simulink model "FinalSim"  (R2022b)
settings: Solver=VariableStepAuto  StartTime=0.0  StopTime=10  RelTol=1e-3
libraries: eeGeneralControl x3
(part 5 of 7)

== system FinalSim/Shoulder Adductor Model/Shoulder Transverse Flexors1/fascicles (CE & PE)/Type S Motor Units ==
  fenv : Inport
  V,L : Inport  Port=2
  Fpe2 : Inport  Port=3
  1/Ty : Gain  Gain=5  SaturateOnIntegerOverflow=on  OutDataTypeStr=Inherit: Same as input  ParamDataTypeStr=Inherit: Same as input
  Af*(FL*FV+PE2) : Product  InputSameDT=on  RndMeth=Zero  SaturateOnIntegerOverflow=on  OutDataTypeStr=Inherit: Same as first input
  Demux all Units : Demux  Outputs=2
      settings: DisplayOption=none
  FL : Fcn  Expr=exp(-abs((u^2.3-1)/1.1244)^1.62)
  FL*FV : Product  InputSameDT=on  RndMeth=Zero  SaturateOnIntegerOverflow=on  OutDataTypeStr=Inherit: Same as first input
  FV (lengthen) : Fcn  Expr=(0.34936-(-4.7+8.41*u(2)+-5.31*u(2)^2)*u(1))/(0.34936+u(1))
  FV (shorten) : Fcn  Expr=(-7.88-u(1))/(-7.88+(5.88+0*u(2))*u(1))
  Motor Unit 1 : Subsystem
  Motor Unit 2 : Subsystem
  PCSA 1 : Gain  Gain=0.21429  SaturateOnIntegerOverflow=on  OutDataTypeStr=Inherit: Same as input  ParamDataTypeStr=Inherit: Same as input
  PCSA 2 : Gain  Gain=0.28571  SaturateOnIntegerOverflow=on  OutDataTypeStr=Inherit: Same as input  ParamDataTypeStr=Inherit: Same as input
  PE+FL*FV : Sum  InputSameDT=on  SaturateOnIntegerOverflow=on  OutDataTypeStr=Inherit: Same as first input
  Sum all Units : Sum  InputSameDT=on  SaturateOnIntegerOverflow=on  OutDataTypeStr=Inherit: Same as first input
  Y,L : Mux  Inputs=2
  newY-oldY : Sum  Inputs=+-  InputSameDT=on  SaturateOnIntegerOverflow=on  OutDataTypeStr=Inherit: Same as first input
  split V,L : Demux  Outputs=2
      settings: DisplayOption=none
  v > 0? : Switch
  y'->y : Integrator  InitialCondition=1
  yield : Fcn  Expr=1-0.35*(1-exp(-abs(u)/0.1))
  F (Fo) : Outport
  wires:
  split V,L/1 -> yield/1, v > 0?/2
  yield/1 -> newY-oldY/1
  newY-oldY/1 -> 1/Ty/1
  1/Ty/1 -> y'->y/1
  y'->y/1 -> newY-oldY/2, Y,L/1
  Y,L/1 -> Motor Unit 1/2(Y,L), Motor Unit 2/2(Y,L)
  Demux all Units/1 -> Motor Unit 1/1(fenv)
  Motor Unit 1/1(A) -> PCSA 1/1
  PCSA 1/1 -> Sum all Units/1
  Demux all Units/2 -> Motor Unit 2/1(fenv)
  Motor Unit 2/1(A) -> PCSA 2/1
  PCSA 2/1 -> Sum all Units/2
  Fpe2/1 -> PE+FL*FV/1
  V,L/1 -> FV (lengthen)/1, FV (shorten)/1, split V,L/1
  FV (lengthen)/1 -> v > 0?/1
  FV (shorten)/1 -> v > 0?/3
  split V,L/2 -> FL/1, Y,L/2
  FL/1 -> FL*FV/2
  v > 0?/1 -> FL*FV/1
  FL*FV/1 -> PE+FL*FV/2
  PE+FL*FV/1 -> Af*(FL*FV+PE2)/1
  fenv/1 -> Demux all Units/1
  Sum all Units/1 -> Af*(FL*FV+PE2)/2
  Af*(FL*FV+PE2)/1 -> F (Fo)/1

== system FinalSim/Shoulder Extensor/fascicles (CE & PE)/Type F Motor Units/Motor Unit 1 ==
  fenv : Inport
  Y,L : Inport  Port=2
  1/Tf (feff' < 0) : Fcn  Expr=u(2)/(0.02822+0.01513*u(3))
  1/Tf (feff' > 0) : Fcn  Expr=1/(0.02057*u(2)^2+0.0136*u(4))
  1/Ts : Gain  Gain=23.2558  SaturateOnIntegerOverflow=on  OutDataTypeStr=Inherit: Same as input  ParamDataTypeStr=Inherit: Same as input
  Af : Fcn  Expr=1-exp(-(u(1)*u(4)*u(3)/(0.56*u(2)))^u(2))
  Leff' : Fcn  Expr=(u(2)-u(1))^3/((1-u(3))*8.8e-005)
  Leff'->Leff : Integrator  InitialCondition=1
  "Leff,L, Af,fenv" : Mux
  S and old S diff : Sum  Inputs=-+  InputSameDT=on  SaturateOnIntegerOverflow=on  OutDataTypeStr=Inherit: Same as first input
  Y,nf,feff,S : Mux
  aS1 : Constant  Value=1.76
  aS2 : Constant  Value=0.96
  demux Y,L : Demux  Outputs=2
      settings: DisplayOption=none
  feff' : Product  InputSameDT=on  RndMeth=Zero  SaturateOnIntegerOverflow=on  OutDataTypeStr=Inherit: Same as first input
  feff' > 0? : Switch
  feff'->feff : Integrator
  feff>0.1? : Switch  Threshold=0.1
  fenv-fint : Sum  Inputs=+-  InputSameDT=on  SaturateOnIntegerOverflow=on  OutDataTypeStr=Inherit: Same as first input
  fint' : Product  InputSameDT=on  RndMeth=Zero  SaturateOnIntegerOverflow=on  OutDataTypeStr=Inherit: Same as first input
  fint'->fint : Integrator
  fint-feff : Sum  Inputs=+-  InputSameDT=on  SaturateOnIntegerOverflow=on  OutDataTypeStr=Inherit: Same as first input
  nf : Fcn  Expr=2.11+3.31*(1/u-1)
  s'->s : Integrator  InitialCondition=1.76
  A : Outport
  wires:
  Y,L/1 -> demux Y,L/1
  demux Y,L/1 -> Y,nf,feff,S/1
  demux Y,L/2 -> "Leff,L, Af,fenv"/2
  "Leff,L, Af,fenv"/1 -> 1/Tf (feff' < 0)/1, Leff'/1, 1/Tf (feff' > 0)/1
  1/Tf (feff' > 0)/1 -> feff' > 0?/1
  1/Tf (feff' < 0)/1 -> feff' > 0?/3
  fenv/1 -> fenv-fint/1, "Leff,L, Af,fenv"/4
  fenv-fint/1 -> fint'/2
  fint'/1 -> fint'->fint/1
  fint'->fint/1 -> fint-feff/1, fenv-fint/2
  fint-feff/1 -> feff'/2, feff' > 0?/2
  feff' > 0?/1 -> feff'/1, fint'/1
  feff'/1 -> feff'->feff/1
  feff'->feff/1 -> fint-feff/2, Y,nf,feff,S/3, feff>0.1?/2
  Y,nf,feff,S/1 -> Af/1
  Af/1 -> "Leff,L, Af,fenv"/3, A/1
  Leff'/1 -> Leff'->Leff/1
  Leff'->Leff/1 -> "Leff,L, Af,fenv"/1, nf/1
  nf/1 -> Y,nf,feff,S/2
  aS2/1 -> feff>0.1?/1
  aS1/1 -> feff>0.1?/3
  feff>0.1?/1 -> S and old S diff/2
  S and old S diff/1 -> 1/Ts/1
  1/Ts/1 -> s'->s/1
  s'->s/1 -> S and old S diff/1, Y,nf,feff,S/4

== system FinalSim/Shoulder Extensor/fascicles (CE & PE)/Type F Motor Units/Motor Unit 2 ==
  fenv : Inport
  Y,L : Inport  Port=2
  1/Tf (feff' < 0) : Fcn  Expr=u(2)/(0.02822+0.01513*u(3))
  1/Tf (feff' > 0) : Fcn  Expr=1/(0.02057*u(2)^2+0.0136*u(4))
  1/Ts : Gain  Gain=23.2558  SaturateOnIntegerOverflow=on  OutDataTypeStr=Inherit: Same as input  ParamDataTypeStr=Inherit: Same as input
  Af : Fcn  Expr=1-exp(-(u(1)*u(4)*u(3)/(0.56*u(2)))^u(2))
  Leff' : Fcn  Expr=(u(2)-u(1))^3/((1-u(3))*8.8e-005)
  Leff'->Leff : Integrator  InitialCondition=1
  "Leff,L, Af,fenv" : Mux
  S and old S diff : Sum  Inputs=-+  InputSameDT=on  SaturateOnIntegerOverflow=on  OutDataTypeStr=Inherit: Same as first input
  Y,nf,feff,S : Mux
  aS1 : Constant  Value=1.76
  aS2 : Constant  Value=0.96
  demux Y,L : Demux  Outputs=2
      settings: DisplayOption=none
  feff' : Product  InputSameDT=on  RndMeth=Zero  SaturateOnIntegerOverflow=on  OutDataTypeStr=Inherit: Same as first input
  feff' > 0? : Switch
  feff'->feff : Integrator
  feff>0.1? : Switch  Threshold=0.1
  fenv-fint : Sum  Inputs=+-  InputSameDT=on  SaturateOnIntegerOverflow=on  OutDataTypeStr=Inherit: Same as first input
  fint' : Product  InputSameDT=on  RndMeth=Zero  SaturateOnIntegerOverflow=on  OutDataTypeStr=Inherit: Same as first input
  fint'->fint : Integrator
  fint-feff : Sum  Inputs=+-  InputSameDT=on  SaturateOnIntegerOverflow=on  OutDataTypeStr=Inherit: Same as first input
  nf : Fcn  Expr=2.11+3.31*(1/u-1)
  s'->s : Integrator  InitialCondition=1.76
  A : Outport
  wires:
  Y,L/1 -> demux Y,L/1
  demux Y,L/1 -> Y,nf,feff,S/1
  demux Y,L/2 -> "Leff,L, Af,fenv"/2
  "Leff,L, Af,fenv"/1 -> 1/Tf (feff' < 0)/1, Leff'/1, 1/Tf (feff' > 0)/1
  1/Tf (feff' > 0)/1 -> feff' > 0?/1
  1/Tf (feff' < 0)/1 -> feff' > 0?/3
  fenv/1 -> fenv-fint/1, "Leff,L, Af,fenv"/4
  fenv-fint/1 -> fint'/2
  fint'/1 -> fint'->fint/1
  fint'->fint/1 -> fint-feff/1, fenv-fint/2
  fint-feff/1 -> feff'/2, feff' > 0?/2
  feff' > 0?/1 -> feff'/1, fint'/1
  feff'/1 -> feff'->feff/1
  feff'->feff/1 -> fint-feff/2, Y,nf,feff,S/3, feff>0.1?/2
  Y,nf,feff,S/1 -> Af/1
  Af/1 -> "Leff,L, Af,fenv"/3, A/1
  Leff'/1 -> Leff'->Leff/1
  Leff'->Leff/1 -> "Leff,L, Af,fenv"/1, nf/1
  nf/1 -> Y,nf,feff,S/2
  aS2/1 -> feff>0.1?/1
  aS1/1 -> feff>0.1?/3
  feff>0.1?/1 -> S and old S diff/2
  S and old S diff/1 -> 1/Ts/1
  1/Ts/1 -> s'->s/1
  s'->s/1 -> S and old S diff/1, Y,nf,feff,S/4

== system FinalSim/Shoulder Extensor/fascicles (CE & PE)/Type F Motor Units/Motor Unit 3 ==
  fenv : Inport
  Y,L : Inport  Port=2
  1/Tf (feff' < 0) : Fcn  Expr=u(2)/(0.02822+0.01513*u(3))
  1/Tf (feff' > 0) : Fcn  Expr=1/(0.02057*u(2)^2+0.0136*u(4))
  1/Ts : Gain  Gain=23.2558  SaturateOnIntegerOverflow=on  OutDataTypeStr=Inherit: Same as input  ParamDataTypeStr=Inherit: Same as input
  Af : Fcn  Expr=1-exp(-(u(1)*u(4)*u(3)/(0.56*u(2)))^u(2))
  Leff' : Fcn  Expr=(u(2)-u(1))^3/((1-u(3))*8.8e-005)
  Leff'->Leff : Integrator  InitialCondition=1
  "Leff,L, Af,fenv" : Mux
  S and old S diff : Sum  Inputs=-+  InputSameDT=on  SaturateOnIntegerOverflow=on  OutDataTypeStr=Inherit: Same as first input
  Y,nf,feff,S : Mux
  aS1 : Constant  Value=1.76
  aS2 : Constant  Value=0.96
  demux Y,L : Demux  Outputs=2
      settings: DisplayOption=none
  feff' : Product  InputSameDT=on  RndMeth=Zero  SaturateOnIntegerOverflow=on  OutDataTypeStr=Inherit: Same as first input
  feff' > 0? : Switch
  feff'->feff : Integrator
  feff>0.1? : Switch  Threshold=0.1
  fenv-fint : Sum  Inputs=+-  InputSameDT=on  SaturateOnIntegerOverflow=on  OutDataTypeStr=Inherit: Same as first input
  fint' : Product  InputSameDT=on  RndMeth=Zero  SaturateOnIntegerOverflow=on  OutDataTypeStr=Inherit: Same as first input
  fint'->fint : Integrator
  fint-feff : Sum  Inputs=+-  InputSameDT=on  SaturateOnIntegerOverflow=on  OutDataTypeStr=Inherit: Same as first input
  nf : Fcn  Expr=2.11+3.31*(1/u-1)
  s'->s : Integrator  InitialCondition=1.76
  A : Outport
  wires:
  Y,L/1 -> demux Y,L/1
  demux Y,L/1 -> Y,nf,feff,S/1
  demux Y,L/2 -> "Leff,L, Af,fenv"/2
  "Leff,L, Af,fenv"/1 -> 1/Tf (feff' < 0)/1, Leff'/1, 1/Tf (feff' > 0)/1
  1/Tf (feff' > 0)/1 -> feff' > 0?/1
  1/Tf (feff' < 0)/1 -> feff' > 0?/3
  fenv/1 -> fenv-fint/1, "Leff,L, Af,fenv"/4
  fenv-fint/1 -> fint'/2
  fint'/1 -> fint'->fint/1
  fint'->fint/1 -> fint-feff/1, fenv-fint/2
  fint-feff/1 -> feff'/2, feff' > 0?/2
  feff' > 0?/1 -> feff'/1, fint'/1
  feff'/1 -> feff'->feff/1
  feff'->feff/1 -> fint-feff/2, Y,nf,feff,S/3, feff>0.1?/2
  Y,nf,feff,S/1 -> Af/1
  Af/1 -> "Leff,L, Af,fenv"/3, A/1
  Leff'/1 -> Leff'->Leff/1
  Leff'->Leff/1 -> "Leff,L, Af,fenv"/1, nf/1
  nf/1 -> Y,nf,feff,S/2
  aS2/1 -> feff>0.1?/1
  aS1/1 -> feff>0.1?/3
  feff>0.1?/1 -> S and old S diff/2
  S and old S diff/1 -> 1/Ts/1
  1/Ts/1 -> s'->s/1
  s'->s/1 -> S and old S diff/1, Y,nf,feff,S/4

== system FinalSim/Shoulder Extensor/fascicles (CE & PE)/Type S Motor Units/Motor Unit 1 ==
  fenv : Inport
  Y,L : Inport  Port=2
  1/Tf (feff' < 0) : Fcn  Expr=u(2)/(0.047033+0.025217*u(3))
  1/Tf (feff' > 0) : Fcn  Expr=1/(0.034283*u(2)^2+0.022667*u(4))
  Af : Fcn  Expr=1-exp(-(u(1)*u(4)*u(3)/(0.56*u(2)))^u(2))
  Leff' : Fcn  Expr=(u(2)-u(1))^3/((1-u(3))*8.8e-005)
  Leff'->Leff : Integrator  InitialCondition=1
  "Leff,L, Af,fenv" : Mux
  Y,nf,feff,S : Mux
  aS : Constant
  demux Y,L : Demux  Outputs=2
      settings: DisplayOption=none
  feff' : Product  InputSameDT=on  RndMeth=Zero  SaturateOnIntegerOverflow=on  OutDataTypeStr=Inherit: Same as first input
  feff' > 0? : Switch
  feff'->feff : Integrator
  fenv-fint : Sum  Inputs=+-  InputSameDT=on  SaturateOnIntegerOverflow=on  OutDataTypeStr=Inherit: Same as first input
  fint' : Product  InputSameDT=on  RndMeth=Zero  SaturateOnIntegerOverflow=on  OutDataTypeStr=Inherit: Same as first input
  fint'->fint : Integrator
  fint-feff : Sum  Inputs=+-  InputSameDT=on  SaturateOnIntegerOverflow=on  OutDataTypeStr=Inherit: Same as first input
  nf : Fcn  Expr=2.11+5*(1/u-1)
  A : Outport
  wires:
  Y,L/1 -> demux Y,L/1
  demux Y,L/1 -> Y,nf,feff,S/1
  demux Y,L/2 -> "Leff,L, Af,fenv"/2
  "Leff,L, Af,fenv"/1 -> 1/Tf (feff' < 0)/1, Leff'/1, 1/Tf (feff' > 0)/1
  1/Tf (feff' > 0)/1 -> feff' > 0?/1
  1/Tf (feff' < 0)/1 -> feff' > 0?/3
  fenv/1 -> fenv-fint/1, "Leff,L, Af,fenv"/4
  fenv-fint/1 -> fint'/2
  fint'/1 -> fint'->fint/1
  fint'->fint/1 -> fint-feff/1, fenv-fint/2
  fint-feff/1 -> feff'/2, feff' > 0?/2
  feff' > 0?/1 -> feff'/1, fint'/1
  feff'/1 -> feff'->feff/1
  feff'->feff/1 -> Y,nf,feff,S/3, fint-feff/2
  Y,nf,feff,S/1 -> Af/1
  Af/1 -> "Leff,L, Af,fenv"/3, A/1
  Leff'/1 -> Leff'->Leff/1
  Leff'->Leff/1 -> "Leff,L, Af,fenv"/1, nf/1
  nf/1 -> Y,nf,feff,S/2
  aS/1 -> Y,nf,feff,S/4

== system FinalSim/Shoulder Extensor/fascicles (CE & PE)/Type S Motor Units/Motor Unit 2 ==
  fenv : Inport
  Y,L : Inport  Port=2
  1/Tf (feff' < 0) : Fcn  Expr=u(2)/(0.047033+0.025217*u(3))
  1/Tf (feff' > 0) : Fcn  Expr=1/(0.034283*u(2)^2+0.022667*u(4))
  Af : Fcn  Expr=1-exp(-(u(1)*u(4)*u(3)/(0.56*u(2)))^u(2))
  Leff' : Fcn  Expr=(u(2)-u(1))^3/((1-u(3))*8.8e-005)
  Leff'->Leff : Integrator  InitialCondition=1
  "Leff,L, Af,fenv" : Mux
  Y,nf,feff,S : Mux
  aS : Constant
  demux Y,L : Demux  Outputs=2
      settings: DisplayOption=none
  feff' : Product  InputSameDT=on  RndMeth=Zero  SaturateOnIntegerOverflow=on  OutDataTypeStr=Inherit: Same as first input
  feff' > 0? : Switch
  feff'->feff : Integrator
  fenv-fint : Sum  Inputs=+-  InputSameDT=on  SaturateOnIntegerOverflow=on  OutDataTypeStr=Inherit: Same as first input
  fint' : Product  InputSameDT=on  RndMeth=Zero  SaturateOnIntegerOverflow=on  OutDataTypeStr=Inherit: Same as first input
  fint'->fint : Integrator
  fint-feff : Sum  Inputs=+-  InputSameDT=on  SaturateOnIntegerOverflow=on  OutDataTypeStr=Inherit: Same as first input
  nf : Fcn  Expr=2.11+5*(1/u-1)
  A : Outport
  wires:
  Y,L/1 -> demux Y,L/1
  demux Y,L/1 -> Y,nf,feff,S/1
  demux Y,L/2 -> "Leff,L, Af,fenv"/2
  "Leff,L, Af,fenv"/1 -> 1/Tf (feff' < 0)/1, Leff'/1, 1/Tf (feff' > 0)/1
  1/Tf (feff' > 0)/1 -> feff' > 0?/1
  1/Tf (feff' < 0)/1 -> feff' > 0?/3
  fenv/1 -> fenv-fint/1, "Leff,L, Af,fenv"/4
  fenv-fint/1 -> fint'/2
  fint'/1 -> fint'->fint/1
  fint'->fint/1 -> fint-feff/1, fenv-fint/2
  fint-feff/1 -> feff'/2, feff' > 0?/2
  feff' > 0?/1 -> feff'/1, fint'/1
  feff'/1 -> feff'->feff/1
  feff'->feff/1 -> Y,nf,feff,S/3, fint-feff/2
  Y,nf,feff,S/1 -> Af/1
  Af/1 -> "Leff,L, Af,fenv"/3, A/1
  Leff'/1 -> Leff'->Leff/1
  Leff'->Leff/1 -> "Leff,L, Af,fenv"/1, nf/1
  nf/1 -> Y,nf,feff,S/2
  aS/1 -> Y,nf,feff,S/4

== system FinalSim/Shoulder Extensor Model/Shoulder Abductors1/Recruitment/Type F Motor Unit 1 ==
  Activation : Inport
  Reached recruitment threshold? : Switch  Threshold=0.50667
  determine frequency : Fcn  Expr=((2-0.5)/(1-(0.50667)))*(u(1)-(0.50667))+0.5
  zero : Constant  Value=0
  Frequency (f0.5) : Outport
  wires:
  Activation/1 -> Reached recruitment threshold?/2, determine frequency/1
  Reached recruitment threshold?/1 -> Frequency (f0.5)/1
  determine frequency/1 -> Reached recruitment threshold?/1
  zero/1 -> Reached recruitment threshold?/3

== system FinalSim/Shoulder Extensor Model/Shoulder Abductors1/Recruitment/Type F Motor Unit 2 ==
  Activation : Inport
  Reached recruitment threshold? : Switch  Threshold=0.64
  determine frequency : Fcn  Expr=((2-0.5)/(1-(0.64)))*(u(1)-(0.64))+0.5
  zero : Constant  Value=0
  Frequency (f0.5) : Outport
  wires:
  Activation/1 -> Reached recruitment threshold?/2, determine frequency/1
  Reached recruitment threshold?/1 -> Frequency (f0.5)/1
  determine frequency/1 -> Reached recruitment threshold?/1
  zero/1 -> Reached recruitment threshold?/3

== system FinalSim/Shoulder Extensor Model/Shoulder Abductors1/Recruitment/Type F Motor Unit 3 ==
  Activation : Inport
  Reached recruitment threshold? : Switch  Threshold=0.8
  determine frequency : Fcn  Expr=((2-0.5)/(1-(0.8)))*(u(1)-(0.8))+0.5
  zero : Constant  Value=0
  Frequency (f0.5) : Outport
  wires:
  Activation/1 -> Reached recruitment threshold?/2, determine frequency/1
  Reached recruitment threshold?/1 -> Frequency (f0.5)/1
  determine frequency/1 -> Reached recruitment threshold?/1
  zero/1 -> Reached recruitment threshold?/3

== system FinalSim/Shoulder Extensor Model/Shoulder Abductors1/Recruitment/Type S Motor Unit 1 ==
  Activation : Inport
  Reached recruitment threshold? : Switch  Threshold=0.17143
  determine frequency : Fcn  Expr=((2-0.5)/(1-(0.17143)))*(u(1)-(0.17143))+0.5
  zero : Constant  Value=0
  Frequency (f0.5) : Outport
  wires:
  Activation/1 -> Reached recruitment threshold?/2, determine frequency/1
  Reached recruitment threshold?/1 -> Frequency (f0.5)/1
  determine frequency/1 -> Reached recruitment threshold?/1
  zero/1 -> Reached recruitment threshold?/3

== system FinalSim/Shoulder Extensor Model/Shoulder Abductors1/Recruitment/Type S Motor Unit 2 ==
  Activation : Inport
  Reached recruitment threshold? : Switch  Threshold=0.4
  determine frequency : Fcn  Expr=((2-0.5)/(1-(0.4)))*(u(1)-(0.4))+0.5
  zero : Constant  Value=0
  Frequency (f0.5) : Outport
  wires:
  Activation/1 -> Reached recruitment threshold?/2, determine frequency/1
  Reached recruitment threshold?/1 -> Frequency (f0.5)/1
  determine frequency/1 -> Reached recruitment threshold?/1
  zero/1 -> Reached recruitment threshold?/3

== system FinalSim/Shoulder Extensor Model/Shoulder Abductors1/fascicles (CE & PE)/Type F Motor Units ==
  fenv : Inport
  V,L : Inport  Port=2
  Fpe2 : Inport  Port=3
  Af*(FL*FV+PE2) : Product  InputSameDT=on  RndMeth=Zero  SaturateOnIntegerOverflow=on  OutDataTypeStr=Inherit: Same as first input
  Constant : Constant
  Demux all Units : Demux  Outputs=3
      settings: DisplayOption=none
  FL : Fcn  Expr=exp(-abs((u^1.55-1)/0.74633)^2.12)
  FL*FV : Product  InputSameDT=on  RndMeth=Zero  SaturateOnIntegerOverflow=on  OutDataTypeStr=Inherit: Same as first input
  FV (lengthen) : Fcn  Expr=(0.68637-(-1.53+0*u(2)+0*u(2)^2)*u(1))/(0.68637+u(1))
  FV (shorten) : Fcn  Expr=(-9.1516-u(1))/(-9.1516+(-5.7+9.18*u(2))*u(1))
  Motor Unit 1 : Subsystem
  Motor Unit 2 : Subsystem
  Motor Unit 3 : Subsystem
  PCSA 1 : Gain  Gain=0.13333  SaturateOnIntegerOverflow=on  OutDataTypeStr=Inherit: Same as input  ParamDataTypeStr=Inherit: Same as input
  PCSA 2 : Gain  Gain=0.16667  SaturateOnIntegerOverflow=on  OutDataTypeStr=Inherit: Same as input  ParamDataTypeStr=Inherit: Same as input
  PCSA 3 : Gain  Gain=0.2  SaturateOnIntegerOverflow=on  OutDataTypeStr=Inherit: Same as input  ParamDataTypeStr=Inherit: Same as input
  PE+FL*FV : Sum  InputSameDT=on  SaturateOnIntegerOverflow=on  OutDataTypeStr=Inherit: Same as first input
  Sum all Units : Sum  Inputs=+++  InputSameDT=on  SaturateOnIntegerOverflow=on  OutDataTypeStr=Inherit: Same as first input
  Y,L : Mux  Inputs=2
  split V,L : Demux  Outputs=2
      settings: DisplayOption=none
  v > 0? : Switch
  F (Fo) : Outport
  wires:
  Constant/1 -> Y,L/1
  Y,L/1 -> Motor Unit 1/2(Y,L), Motor Unit 2/2(Y,L), Motor Unit 3/2(Y,L)
  Demux all Units/1 -> Motor Unit 1/1(fenv)
  Motor Unit 1/1(A) -> PCSA 1/1
  PCSA 1/1 -> Sum all Units/1
  Demux all Units/2 -> Motor Unit 2/1(fenv)
  Motor Unit 2/1(A) -> PCSA 2/1
  PCSA 2/1 -> Sum all Units/2
  Demux all Units/3 -> Motor Unit 3/1(fenv)
  Motor Unit 3/1(A) -> PCSA 3/1
  PCSA 3/1 -> Sum all Units/3
  Fpe2/1 -> PE+FL*FV/1
  V,L/1 -> FV (lengthen)/1, FV (shorten)/1, split V,L/1
  FV (lengthen)/1 -> v > 0?/1
  FV (shorten)/1 -> v > 0?/3
  split V,L/2 -> FL/1, Y,L/2
  FL/1 -> FL*FV/2
  split V,L/1 -> v > 0?/2
  v > 0?/1 -> FL*FV/1
  FL*FV/1 -> PE+FL*FV/2
  PE+FL*FV/1 -> Af*(FL*FV+PE2)/1
  fenv/1 -> Demux all Units/1
  Sum all Units/1 -> Af*(FL*FV+PE2)/2
  Af*(FL*FV+PE2)/1 -> F (Fo)/1

== system FinalSim/Shoulder Extensor Model/Shoulder Abductors1/fascicles (CE & PE)/Type S Motor Units ==
  fenv : Inport
  V,L : Inport  Port=2
  Fpe2 : Inport  Port=3
  1/Ty : Gain  Gain=5  SaturateOnIntegerOverflow=on  OutDataTypeStr=Inherit: Same as input  ParamDataTypeStr=Inherit: Same as input
  Af*(FL*FV+PE2) : Product  InputSameDT=on  RndMeth=Zero  SaturateOnIntegerOverflow=on  OutDataTypeStr=Inherit: Same as first input
  Demux all Units : Demux  Outputs=2
      settings: DisplayOption=none
  FL : Fcn  Expr=exp(-abs((u^2.3-1)/1.1244)^1.62)
  FL*FV : Product  InputSameDT=on  RndMeth=Zero  SaturateOnIntegerOverflow=on  OutDataTypeStr=Inherit: Same as first input
  FV (lengthen) : Fcn  Expr=(0.34936-(-4.7+8.41*u(2)+-5.31*u(2)^2)*u(1))/(0.34936+u(1))
  FV (shorten) : Fcn  Expr=(-7.88-u(1))/(-7.88+(5.88+0*u(2))*u(1))
  Motor Unit 1 : Subsystem
  Motor Unit 2 : Subsystem
  PCSA 1 : Gain  Gain=0.21429  SaturateOnIntegerOverflow=on  OutDataTypeStr=Inherit: Same as input  ParamDataTypeStr=Inherit: Same as input
  PCSA 2 : Gain  Gain=0.28571  SaturateOnIntegerOverflow=on  OutDataTypeStr=Inherit: Same as input  ParamDataTypeStr=Inherit: Same as input
  PE+FL*FV : Sum  InputSameDT=on  SaturateOnIntegerOverflow=on  OutDataTypeStr=Inherit: Same as first input
  Sum all Units : Sum  InputSameDT=on  SaturateOnIntegerOverflow=on  OutDataTypeStr=Inherit: Same as first input
  Y,L : Mux  Inputs=2
  newY-oldY : Sum  Inputs=+-  InputSameDT=on  SaturateOnIntegerOverflow=on  OutDataTypeStr=Inherit: Same as first input
  split V,L : Demux  Outputs=2
      settings: DisplayOption=none
  v > 0? : Switch
  y'->y : Integrator  InitialCondition=1
  yield : Fcn  Expr=1-0.35*(1-exp(-abs(u)/0.1))
  F (Fo) : Outport
  wires:
  split V,L/1 -> yield/1, v > 0?/2
  yield/1 -> newY-oldY/1
  newY-oldY/1 -> 1/Ty/1
  1/Ty/1 -> y'->y/1
  y'->y/1 -> newY-oldY/2, Y,L/1
  Y,L/1 -> Motor Unit 1/2(Y,L), Motor Unit 2/2(Y,L)
  Demux all Units/1 -> Motor Unit 1/1(fenv)
  Motor Unit 1/1(A) -> PCSA 1/1
  PCSA 1/1 -> Sum all Units/1
  Demux all Units/2 -> Motor Unit 2/1(fenv)
  Motor Unit 2/1(A) -> PCSA 2/1
  PCSA 2/1 -> Sum all Units/2
  Fpe2/1 -> PE+FL*FV/1
  V,L/1 -> FV (lengthen)/1, FV (shorten)/1, split V,L/1
  FV (lengthen)/1 -> v > 0?/1
  FV (shorten)/1 -> v > 0?/3
  split V,L/2 -> FL/1, Y,L/2
  FL/1 -> FL*FV/2
  v > 0?/1 -> FL*FV/1
  FL*FV/1 -> PE+FL*FV/2
  PE+FL*FV/1 -> Af*(FL*FV+PE2)/1
  fenv/1 -> Demux all Units/1
  Sum all Units/1 -> Af*(FL*FV+PE2)/2
  Af*(FL*FV+PE2)/1 -> F (Fo)/1

== system FinalSim/Shoulder Flexor/fascicles (CE & PE)/Type F Motor Units/Motor Unit 1 ==
  fenv : Inport
  Y,L : Inport  Port=2
  1/Tf (feff' < 0) : Fcn  Expr=u(2)/(0.02822+0.01513*u(3))
  1/Tf (feff' > 0) : Fcn  Expr=1/(0.02057*u(2)^2+0.0136*u(4))
  1/Ts : Gain  Gain=23.2558  SaturateOnIntegerOverflow=on  OutDataTypeStr=Inherit: Same as input  ParamDataTypeStr=Inherit: Same as input
  Af : Fcn  Expr=1-exp(-(u(1)*u(4)*u(3)/(0.56*u(2)))^u(2))
  Leff' : Fcn  Expr=(u(2)-u(1))^3/((1-u(3))*8.8e-005)
  Leff'->Leff : Integrator  InitialCondition=1
  "Leff,L, Af,fenv" : Mux
  S and old S diff : Sum  Inputs=-+  InputSameDT=on  SaturateOnIntegerOverflow=on  OutDataTypeStr=Inherit: Same as first input
  Y,nf,feff,S : Mux
  aS1 : Constant  Value=1.76
  aS2 : Constant  Value=0.96
  demux Y,L : Demux  Outputs=2
      settings: DisplayOption=none
  feff' : Product  InputSameDT=on  RndMeth=Zero  SaturateOnIntegerOverflow=on  OutDataTypeStr=Inherit: Same as first input
  feff' > 0? : Switch
  feff'->feff : Integrator
  feff>0.1? : Switch  Threshold=0.1
  fenv-fint : Sum  Inputs=+-  InputSameDT=on  SaturateOnIntegerOverflow=on  OutDataTypeStr=Inherit: Same as first input
  fint' : Product  InputSameDT=on  RndMeth=Zero  SaturateOnIntegerOverflow=on  OutDataTypeStr=Inherit: Same as first input
  fint'->fint : Integrator
  fint-feff : Sum  Inputs=+-  InputSameDT=on  SaturateOnIntegerOverflow=on  OutDataTypeStr=Inherit: Same as first input
  nf : Fcn  Expr=2.11+3.31*(1/u-1)
  s'->s : Integrator  InitialCondition=1.76
  A : Outport
  wires:
  Y,L/1 -> demux Y,L/1
  demux Y,L/1 -> Y,nf,feff,S/1
  demux Y,L/2 -> "Leff,L, Af,fenv"/2
  "Leff,L, Af,fenv"/1 -> 1/Tf (feff' < 0)/1, Leff'/1, 1/Tf (feff' > 0)/1
  1/Tf (feff' > 0)/1 -> feff' > 0?/1
  1/Tf (feff' < 0)/1 -> feff' > 0?/3
  fenv/1 -> fenv-fint/1, "Leff,L, Af,fenv"/4
  fenv-fint/1 -> fint'/2
  fint'/1 -> fint'->fint/1
  fint'->fint/1 -> fint-feff/1, fenv-fint/2
  fint-feff/1 -> feff'/2, feff' > 0?/2
  feff' > 0?/1 -> feff'/1, fint'/1
  feff'/1 -> feff'->feff/1
  feff'->feff/1 -> fint-feff/2, Y,nf,feff,S/3, feff>0.1?/2
  Y,nf,feff,S/1 -> Af/1
  Af/1 -> "Leff,L, Af,fenv"/3, A/1
  Leff'/1 -> Leff'->Leff/1
  Leff'->Leff/1 -> "Leff,L, Af,fenv"/1, nf/1
  nf/1 -> Y,nf,feff,S/2
  aS2/1 -> feff>0.1?/1
  aS1/1 -> feff>0.1?/3
  feff>0.1?/1 -> S and old S diff/2
  S and old S diff/1 -> 1/Ts/1
  1/Ts/1 -> s'->s/1
  s'->s/1 -> S and old S diff/1, Y,nf,feff,S/4

== system FinalSim/Shoulder Flexor/fascicles (CE & PE)/Type F Motor Units/Motor Unit 2 ==
  fenv : Inport
  Y,L : Inport  Port=2
  1/Tf (feff' < 0) : Fcn  Expr=u(2)/(0.02822+0.01513*u(3))
  1/Tf (feff' > 0) : Fcn  Expr=1/(0.02057*u(2)^2+0.0136*u(4))
  1/Ts : Gain  Gain=23.2558  SaturateOnIntegerOverflow=on  OutDataTypeStr=Inherit: Same as input  ParamDataTypeStr=Inherit: Same as input
  Af : Fcn  Expr=1-exp(-(u(1)*u(4)*u(3)/(0.56*u(2)))^u(2))
  Leff' : Fcn  Expr=(u(2)-u(1))^3/((1-u(3))*8.8e-005)
  Leff'->Leff : Integrator  InitialCondition=1
  "Leff,L, Af,fenv" : Mux
  S and old S diff : Sum  Inputs=-+  InputSameDT=on  SaturateOnIntegerOverflow=on  OutDataTypeStr=Inherit: Same as first input
  Y,nf,feff,S : Mux
  aS1 : Constant  Value=1.76
  aS2 : Constant  Value=0.96
  demux Y,L : Demux  Outputs=2
      settings: DisplayOption=none
  feff' : Product  InputSameDT=on  RndMeth=Zero  SaturateOnIntegerOverflow=on  OutDataTypeStr=Inherit: Same as first input
  feff' > 0? : Switch
  feff'->feff : Integrator
  feff>0.1? : Switch  Threshold=0.1
  fenv-fint : Sum  Inputs=+-  InputSameDT=on  SaturateOnIntegerOverflow=on  OutDataTypeStr=Inherit: Same as first input
  fint' : Product  InputSameDT=on  RndMeth=Zero  SaturateOnIntegerOverflow=on  OutDataTypeStr=Inherit: Same as first input
  fint'->fint : Integrator
  fint-feff : Sum  Inputs=+-  InputSameDT=on  SaturateOnIntegerOverflow=on  OutDataTypeStr=Inherit: Same as first input
  nf : Fcn  Expr=2.11+3.31*(1/u-1)
  s'->s : Integrator  InitialCondition=1.76
  A : Outport
  wires:
  Y,L/1 -> demux Y,L/1
  demux Y,L/1 -> Y,nf,feff,S/1
  demux Y,L/2 -> "Leff,L, Af,fenv"/2
  "Leff,L, Af,fenv"/1 -> 1/Tf (feff' < 0)/1, Leff'/1, 1/Tf (feff' > 0)/1
  1/Tf (feff' > 0)/1 -> feff' > 0?/1
  1/Tf (feff' < 0)/1 -> feff' > 0?/3
  fenv/1 -> fenv-fint/1, "Leff,L, Af,fenv"/4
  fenv-fint/1 -> fint'/2
  fint'/1 -> fint'->fint/1
  fint'->fint/1 -> fint-feff/1, fenv-fint/2
  fint-feff/1 -> feff'/2, feff' > 0?/2
  feff' > 0?/1 -> feff'/1, fint'/1
  feff'/1 -> feff'->feff/1
  feff'->feff/1 -> fint-feff/2, Y,nf,feff,S/3, feff>0.1?/2
  Y,nf,feff,S/1 -> Af/1
  Af/1 -> "Leff,L, Af,fenv"/3, A/1
  Leff'/1 -> Leff'->Leff/1
  Leff'->Leff/1 -> "Leff,L, Af,fenv"/1, nf/1
  nf/1 -> Y,nf,feff,S/2
  aS2/1 -> feff>0.1?/1
  aS1/1 -> feff>0.1?/3
  feff>0.1?/1 -> S and old S diff/2
  S and old S diff/1 -> 1/Ts/1
  1/Ts/1 -> s'->s/1
  s'->s/1 -> S and old S diff/1, Y,nf,feff,S/4

== system FinalSim/Shoulder Flexor/fascicles (CE & PE)/Type F Motor Units/Motor Unit 3 ==
  fenv : Inport
  Y,L : Inport  Port=2
  1/Tf (feff' < 0) : Fcn  Expr=u(2)/(0.02822+0.01513*u(3))
  1/Tf (feff' > 0) : Fcn  Expr=1/(0.02057*u(2)^2+0.0136*u(4))
  1/Ts : Gain  Gain=23.2558  SaturateOnIntegerOverflow=on  OutDataTypeStr=Inherit: Same as input  ParamDataTypeStr=Inherit: Same as input
  Af : Fcn  Expr=1-exp(-(u(1)*u(4)*u(3)/(0.56*u(2)))^u(2))
  Leff' : Fcn  Expr=(u(2)-u(1))^3/((1-u(3))*8.8e-005)
  Leff'->Leff : Integrator  InitialCondition=1
  "Leff,L, Af,fenv" : Mux
  S and old S diff : Sum  Inputs=-+  InputSameDT=on  SaturateOnIntegerOverflow=on  OutDataTypeStr=Inherit: Same as first input
  Y,nf,feff,S : Mux
  aS1 : Constant  Value=1.76
  aS2 : Constant  Value=0.96
  demux Y,L : Demux  Outputs=2
      settings: DisplayOption=none
  feff' : Product  InputSameDT=on  RndMeth=Zero  SaturateOnIntegerOverflow=on  OutDataTypeStr=Inherit: Same as first input
  feff' > 0? : Switch
  feff'->feff : Integrator
  feff>0.1? : Switch  Threshold=0.1
  fenv-fint : Sum  Inputs=+-  InputSameDT=on  SaturateOnIntegerOverflow=on  OutDataTypeStr=Inherit: Same as first input
  fint' : Product  InputSameDT=on  RndMeth=Zero  SaturateOnIntegerOverflow=on  OutDataTypeStr=Inherit: Same as first input
  fint'->fint : Integrator
  fint-feff : Sum  Inputs=+-  InputSameDT=on  SaturateOnIntegerOverflow=on  OutDataTypeStr=Inherit: Same as first input
  nf : Fcn  Expr=2.11+3.31*(1/u-1)
  s'->s : Integrator  InitialCondition=1.76
  A : Outport
  wires:
  Y,L/1 -> demux Y,L/1
  demux Y,L/1 -> Y,nf,feff,S/1
  demux Y,L/2 -> "Leff,L, Af,fenv"/2
  "Leff,L, Af,fenv"/1 -> 1/Tf (feff' < 0)/1, Leff'/1, 1/Tf (feff' > 0)/1
  1/Tf (feff' > 0)/1 -> feff' > 0?/1
  1/Tf (feff' < 0)/1 -> feff' > 0?/3
  fenv/1 -> fenv-fint/1, "Leff,L, Af,fenv"/4
  fenv-fint/1 -> fint'/2
  fint'/1 -> fint'->fint/1
  fint'->fint/1 -> fint-feff/1, fenv-fint/2
  fint-feff/1 -> feff'/2, feff' > 0?/2
  feff' > 0?/1 -> feff'/1, fint'/1
  feff'/1 -> feff'->feff/1
  feff'->feff/1 -> fint-feff/2, Y,nf,feff,S/3, feff>0.1?/2
  Y,nf,feff,S/1 -> Af/1
  Af/1 -> "Leff,L, Af,fenv"/3, A/1
  Leff'/1 -> Leff'->Leff/1
  Leff'->Leff/1 -> "Leff,L, Af,fenv"/1, nf/1
  nf/1 -> Y,nf,feff,S/2
  aS2/1 -> feff>0.1?/1
  aS1/1 -> feff>0.1?/3
  feff>0.1?/1 -> S and old S diff/2
  S and old S diff/1 -> 1/Ts/1
  1/Ts/1 -> s'->s/1
  s'->s/1 -> S and old S diff/1, Y,nf,feff,S/4

== system FinalSim/Shoulder Flexor/fascicles (CE & PE)/Type S Motor Units/Motor Unit 1 ==
  fenv : Inport
  Y,L : Inport  Port=2
  1/Tf (feff' < 0) : Fcn  Expr=u(2)/(0.047033+0.025217*u(3))
  1/Tf (feff' > 0) : Fcn  Expr=1/(0.034283*u(2)^2+0.022667*u(4))
  Af : Fcn  Expr=1-exp(-(u(1)*u(4)*u(3)/(0.56*u(2)))^u(2))
  Leff' : Fcn  Expr=(u(2)-u(1))^3/((1-u(3))*8.8e-005)
  Leff'->Leff : Integrator  InitialCondition=1
  "Leff,L, Af,fenv" : Mux
  Y,nf,feff,S : Mux
  aS : Constant
  demux Y,L : Demux  Outputs=2
      settings: DisplayOption=none
  feff' : Product  InputSameDT=on  RndMeth=Zero  SaturateOnIntegerOverflow=on  OutDataTypeStr=Inherit: Same as first input
  feff' > 0? : Switch
  feff'->feff : Integrator
  fenv-fint : Sum  Inputs=+-  InputSameDT=on  SaturateOnIntegerOverflow=on  OutDataTypeStr=Inherit: Same as first input
  fint' : Product  InputSameDT=on  RndMeth=Zero  SaturateOnIntegerOverflow=on  OutDataTypeStr=Inherit: Same as first input
  fint'->fint : Integrator
  fint-feff : Sum  Inputs=+-  InputSameDT=on  SaturateOnIntegerOverflow=on  OutDataTypeStr=Inherit: Same as first input
  nf : Fcn  Expr=2.11+5*(1/u-1)
  A : Outport
  wires:
  Y,L/1 -> demux Y,L/1
  demux Y,L/1 -> Y,nf,feff,S/1
  demux Y,L/2 -> "Leff,L, Af,fenv"/2
  "Leff,L, Af,fenv"/1 -> 1/Tf (feff' < 0)/1, Leff'/1, 1/Tf (feff' > 0)/1
  1/Tf (feff' > 0)/1 -> feff' > 0?/1
  1/Tf (feff' < 0)/1 -> feff' > 0?/3
  fenv/1 -> fenv-fint/1, "Leff,L, Af,fenv"/4
  fenv-fint/1 -> fint'/2
  fint'/1 -> fint'->fint/1
  fint'->fint/1 -> fint-feff/1, fenv-fint/2
  fint-feff/1 -> feff'/2, feff' > 0?/2
  feff' > 0?/1 -> feff'/1, fint'/1
  feff'/1 -> feff'->feff/1
  feff'->feff/1 -> Y,nf,feff,S/3, fint-feff/2
  Y,nf,feff,S/1 -> Af/1
  Af/1 -> "Leff,L, Af,fenv"/3, A/1
  Leff'/1 -> Leff'->Leff/1
  Leff'->Leff/1 -> "Leff,L, Af,fenv"/1, nf/1
  nf/1 -> Y,nf,feff,S/2
  aS/1 -> Y,nf,feff,S/4

== system FinalSim/Shoulder Flexor/fascicles (CE & PE)/Type S Motor Units/Motor Unit 2 ==
  fenv : Inport
  Y,L : Inport  Port=2
  1/Tf (feff' < 0) : Fcn  Expr=u(2)/(0.047033+0.025217*u(3))
  1/Tf (feff' > 0) : Fcn  Expr=1/(0.034283*u(2)^2+0.022667*u(4))
  Af : Fcn  Expr=1-exp(-(u(1)*u(4)*u(3)/(0.56*u(2)))^u(2))
  Leff' : Fcn  Expr=(u(2)-u(1))^3/((1-u(3))*8.8e-005)
  Leff'->Leff : Integrator  InitialCondition=1
  "Leff,L, Af,fenv" : Mux
  Y,nf,feff,S : Mux
  aS : Constant
  demux Y,L : Demux  Outputs=2
      settings: DisplayOption=none
  feff' : Product  InputSameDT=on  RndMeth=Zero  SaturateOnIntegerOverflow=on  OutDataTypeStr=Inherit: Same as first input
  feff' > 0? : Switch
  feff'->feff : Integrator
  fenv-fint : Sum  Inputs=+-  InputSameDT=on  SaturateOnIntegerOverflow=on  OutDataTypeStr=Inherit: Same as first input
  fint' : Product  InputSameDT=on  RndMeth=Zero  SaturateOnIntegerOverflow=on  OutDataTypeStr=Inherit: Same as first input
  fint'->fint : Integrator
  fint-feff : Sum  Inputs=+-  InputSameDT=on  SaturateOnIntegerOverflow=on  OutDataTypeStr=Inherit: Same as first input
  nf : Fcn  Expr=2.11+5*(1/u-1)
  A : Outport
  wires:
  Y,L/1 -> demux Y,L/1
  demux Y,L/1 -> Y,nf,feff,S/1
  demux Y,L/2 -> "Leff,L, Af,fenv"/2
  "Leff,L, Af,fenv"/1 -> 1/Tf (feff' < 0)/1, Leff'/1, 1/Tf (feff' > 0)/1
  1/Tf (feff' > 0)/1 -> feff' > 0?/1
  1/Tf (feff' < 0)/1 -> feff' > 0?/3
  fenv/1 -> fenv-fint/1, "Leff,L, Af,fenv"/4
  fenv-fint/1 -> fint'/2
  fint'/1 -> fint'->fint/1
  fint'->fint/1 -> fint-feff/1, fenv-fint/2
  fint-feff/1 -> feff'/2, feff' > 0?/2
  feff' > 0?/1 -> feff'/1, fint'/1
  feff'/1 -> feff'->feff/1
  feff'->feff/1 -> Y,nf,feff,S/3, fint-feff/2
  Y,nf,feff,S/1 -> Af/1
  Af/1 -> "Leff,L, Af,fenv"/3, A/1
  Leff'/1 -> Leff'->Leff/1
  Leff'->Leff/1 -> "Leff,L, Af,fenv"/1, nf/1
  nf/1 -> Y,nf,feff,S/2
  aS/1 -> Y,nf,feff,S/4

== system FinalSim/Shoulder Transverse Model/Shoulder Transverse Flexors1/Recruitment/Type F Motor Unit 1 ==
  Activation : Inport
  Reached recruitment threshold? : Switch  Threshold=0.50667
  determine frequency : Fcn  Expr=((2-0.5)/(1-(0.50667)))*(u(1)-(0.50667))+0.5
  zero : Constant  Value=0
  Frequency (f0.5) : Outport
  wires:
  Activation/1 -> Reached recruitment threshold?/2, determine frequency/1
  Reached recruitment threshold?/1 -> Frequency (f0.5)/1
  determine frequency/1 -> Reached recruitment threshold?/1
  zero/1 -> Reached recruitment threshold?/3

== system FinalSim/Shoulder Transverse Model/Shoulder Transverse Flexors1/Recruitment/Type F Motor Unit 2 ==
  Activation : Inport
  Reached recruitment threshold? : Switch  Threshold=0.64
  determine frequency : Fcn  Expr=((2-0.5)/(1-(0.64)))*(u(1)-(0.64))+0.5
  zero : Constant  Value=0
  Frequency (f0.5) : Outport
  wires:
  Activation/1 -> Reached recruitment threshold?/2, determine frequency/1
  Reached recruitment threshold?/1 -> Frequency (f0.5)/1
  determine frequency/1 -> Reached recruitment threshold?/1
  zero/1 -> Reached recruitment threshold?/3

== system FinalSim/Shoulder Transverse Model/Shoulder Transverse Flexors1/Recruitment/Type F Motor Unit 3 ==
  Activation : Inport
  Reached recruitment threshold? : Switch  Threshold=0.8
  determine frequency : Fcn  Expr=((2-0.5)/(1-(0.8)))*(u(1)-(0.8))+0.5
  zero : Constant  Value=0
  Frequency (f0.5) : Outport
  wires:
  Activation/1 -> Reached recruitment threshold?/2, determine frequency/1
  Reached recruitment threshold?/1 -> Frequency (f0.5)/1
  determine frequency/1 -> Reached recruitment threshold?/1
  zero/1 -> Reached recruitment threshold?/3

== system FinalSim/Shoulder Transverse Model/Shoulder Transverse Flexors1/Recruitment/Type S Motor Unit 1 ==
  Activation : Inport
  Reached recruitment threshold? : Switch  Threshold=0.17143
  determine frequency : Fcn  Expr=((2-0.5)/(1-(0.17143)))*(u(1)-(0.17143))+0.5
  zero : Constant  Value=0
  Frequency (f0.5) : Outport
  wires:
  Activation/1 -> Reached recruitment threshold?/2, determine frequency/1
  Reached recruitment threshold?/1 -> Frequency (f0.5)/1
  determine frequency/1 -> Reached recruitment threshold?/1
  zero/1 -> Reached recruitment threshold?/3

== system FinalSim/Shoulder Transverse Model/Shoulder Transverse Flexors1/Recruitment/Type S Motor Unit 2 ==
  Activation : Inport
  Reached recruitment threshold? : Switch  Threshold=0.4
  determine frequency : Fcn  Expr=((2-0.5)/(1-(0.4)))*(u(1)-(0.4))+0.5
  zero : Constant  Value=0
  Frequency (f0.5) : Outport
  wires:
  Activation/1 -> Reached recruitment threshold?/2, determine frequency/1
  Reached recruitment threshold?/1 -> Frequency (f0.5)/1
  determine frequency/1 -> Reached recruitment threshold?/1
  zero/1 -> Reached recruitment threshold?/3

== system FinalSim/Shoulder Transverse Model/Shoulder Transverse Flexors1/fascicles (CE & PE)/Type F Motor Units ==
  fenv : Inport
  V,L : Inport  Port=2
  Fpe2 : Inport  Port=3
  Af*(FL*FV+PE2) : Product  InputSameDT=on  RndMeth=Zero  SaturateOnIntegerOverflow=on  OutDataTypeStr=Inherit: Same as first input
  Constant : Constant
  Demux all Units : Demux  Outputs=3
      settings: DisplayOption=none
  FL : Fcn  Expr=exp(-abs((u^1.55-1)/0.74633)^2.12)
  FL*FV : Product  InputSameDT=on  RndMeth=Zero  SaturateOnIntegerOverflow=on  OutDataTypeStr=Inherit: Same as first input
  FV (lengthen) : Fcn  Expr=(0.68637-(-1.53+0*u(2)+0*u(2)^2)*u(1))/(0.68637+u(1))
  FV (shorten) : Fcn  Expr=(-9.1516-u(1))/(-9.1516+(-5.7+9.18*u(2))*u(1))
  Motor Unit 1 : Subsystem
  Motor Unit 2 : Subsystem
  Motor Unit 3 : Subsystem
  PCSA 1 : Gain  Gain=0.13333  SaturateOnIntegerOverflow=on  OutDataTypeStr=Inherit: Same as input  ParamDataTypeStr=Inherit: Same as input
  PCSA 2 : Gain  Gain=0.16667  SaturateOnIntegerOverflow=on  OutDataTypeStr=Inherit: Same as input  ParamDataTypeStr=Inherit: Same as input
  PCSA 3 : Gain  Gain=0.2  SaturateOnIntegerOverflow=on  OutDataTypeStr=Inherit: Same as input  ParamDataTypeStr=Inherit: Same as input
  PE+FL*FV : Sum  InputSameDT=on  SaturateOnIntegerOverflow=on  OutDataTypeStr=Inherit: Same as first input
  Sum all Units : Sum  Inputs=+++  InputSameDT=on  SaturateOnIntegerOverflow=on  OutDataTypeStr=Inherit: Same as first input
  Y,L : Mux  Inputs=2
  split V,L : Demux  Outputs=2
      settings: DisplayOption=none
  v > 0? : Switch
  F (Fo) : Outport
  wires:
  Constant/1 -> Y,L/1
  Y,L/1 -> Motor Unit 1/2(Y,L), Motor Unit 2/2(Y,L), Motor Unit 3/2(Y,L)
  Demux all Units/1 -> Motor Unit 1/1(fenv)
  Motor Unit 1/1(A) -> PCSA 1/1
  PCSA 1/1 -> Sum all Units/1
  Demux all Units/2 -> Motor Unit 2/1(fenv)
  Motor Unit 2/1(A) -> PCSA 2/1
  PCSA 2/1 -> Sum all Units/2
  Demux all Units/3 -> Motor Unit 3/1(fenv)
  Motor Unit 3/1(A) -> PCSA 3/1
  PCSA 3/1 -> Sum all Units/3
  Fpe2/1 -> PE+FL*FV/1
  V,L/1 -> FV (lengthen)/1, FV (shorten)/1, split V,L/1
  FV (lengthen)/1 -> v > 0?/1
  FV (shorten)/1 -> v > 0?/3
  split V,L/2 -> FL/1, Y,L/2
  FL/1 -> FL*FV/2
  split V,L/1 -> v > 0?/2
  v > 0?/1 -> FL*FV/1
  FL*FV/1 -> PE+FL*FV/2
  PE+FL*FV/1 -> Af*(FL*FV+PE2)/1
  fenv/1 -> Demux all Units/1
  Sum all Units/1 -> Af*(FL*FV+PE2)/2
  Af*(FL*FV+PE2)/1 -> F (Fo)/1

== system FinalSim/Shoulder Transverse Model/Shoulder Transverse Flexors1/fascicles (CE & PE)/Type S Motor Units ==
  fenv : Inport
  V,L : Inport  Port=2
  Fpe2 : Inport  Port=3
  1/Ty : Gain  Gain=5  SaturateOnIntegerOverflow=on  OutDataTypeStr=Inherit: Same as input  ParamDataTypeStr=Inherit: Same as input
  Af*(FL*FV+PE2) : Product  InputSameDT=on  RndMeth=Zero  SaturateOnIntegerOverflow=on  OutDataTypeStr=Inherit: Same as first input
  Demux all Units : Demux  Outputs=2
      settings: DisplayOption=none
  FL : Fcn  Expr=exp(-abs((u^2.3-1)/1.1244)^1.62)
  FL*FV : Product  InputSameDT=on  RndMeth=Zero  SaturateOnIntegerOverflow=on  OutDataTypeStr=Inherit: Same as first input
  FV (lengthen) : Fcn  Expr=(0.34936-(-4.7+8.41*u(2)+-5.31*u(2)^2)*u(1))/(0.34936+u(1))
  FV (shorten) : Fcn  Expr=(-7.88-u(1))/(-7.88+(5.88+0*u(2))*u(1))
  Motor Unit 1 : Subsystem
  Motor Unit 2 : Subsystem
  PCSA 1 : Gain  Gain=0.21429  SaturateOnIntegerOverflow=on  OutDataTypeStr=Inherit: Same as input  ParamDataTypeStr=Inherit: Same as input
  PCSA 2 : Gain  Gain=0.28571  SaturateOnIntegerOverflow=on  OutDataTypeStr=Inherit: Same as input  ParamDataTypeStr=Inherit: Same as input
  PE+FL*FV : Sum  InputSameDT=on  SaturateOnIntegerOverflow=on  OutDataTypeStr=Inherit: Same as first input
  Sum all Units : Sum  InputSameDT=on  SaturateOnIntegerOverflow=on  OutDataTypeStr=Inherit: Same as first input
  Y,L : Mux  Inputs=2
  newY-oldY : Sum  Inputs=+-  InputSameDT=on  SaturateOnIntegerOverflow=on  OutDataTypeStr=Inherit: Same as first input
  split V,L : Demux  Outputs=2
      settings: DisplayOption=none
  v > 0? : Switch
  y'->y : Integrator  InitialCondition=1
  yield : Fcn  Expr=1-0.35*(1-exp(-abs(u)/0.1))
  F (Fo) : Outport
  wires:
  split V,L/1 -> yield/1, v > 0?/2
  yield/1 -> newY-oldY/1
  newY-oldY/1 -> 1/Ty/1
  1/Ty/1 -> y'->y/1
  y'->y/1 -> newY-oldY/2, Y,L/1
  Y,L/1 -> Motor Unit 1/2(Y,L), Motor Unit 2/2(Y,L)
  Demux all Units/1 -> Motor Unit 1/1(fenv)
  Motor Unit 1/1(A) -> PCSA 1/1
  PCSA 1/1 -> Sum all Units/1
  Demux all Units/2 -> Motor Unit 2/1(fenv)
  Motor Unit 2/1(A) -> PCSA 2/1
  PCSA 2/1 -> Sum all Units/2
  Fpe2/1 -> PE+FL*FV/1
  V,L/1 -> FV (lengthen)/1, FV (shorten)/1, split V,L/1
  FV (lengthen)/1 -> v > 0?/1
  FV (shorten)/1 -> v > 0?/3
  split V,L/2 -> FL/1, Y,L/2
  FL/1 -> FL*FV/2
  v > 0?/1 -> FL*FV/1
  FL*FV/1 -> PE+FL*FV/2
  PE+FL*FV/1 -> Af*(FL*FV+PE2)/1
  fenv/1 -> Demux all Units/1
  Sum all Units/1 -> Af*(FL*FV+PE2)/2
  Af*(FL*FV+PE2)/1 -> F (Fo)/1

== system FinalSim/Tricep Model/Tricep Group/Recruitment/Type F Motor Unit 1 ==
  Activation : Inport
  Reached recruitment threshold? : Switch  Threshold=0.50667
  determine frequency : Fcn  Expr=((2-0.5)/(1-(0.50667)))*(u(1)-(0.50667))+0.5
  zero : Constant  Value=0
  Frequency (f0.5) : Outport
  wires:
  Activation/1 -> Reached recruitment threshold?/2, determine frequency/1
  Reached recruitment threshold?/1 -> Frequency (f0.5)/1
  determine frequency/1 -> Reached recruitment threshold?/1
  zero/1 -> Reached recruitment threshold?/3

== system FinalSim/Tricep Model/Tricep Group/Recruitment/Type F Motor Unit 2 ==
  Activation : Inport
  Reached recruitment threshold? : Switch  Threshold=0.64
  determine frequency : Fcn  Expr=((2-0.5)/(1-(0.64)))*(u(1)-(0.64))+0.5
  zero : Constant  Value=0
  Frequency (f0.5) : Outport
  wires:
  Activation/1 -> Reached recruitment threshold?/2, determine frequency/1
  Reached recruitment threshold?/1 -> Frequency (f0.5)/1
  determine frequency/1 -> Reached recruitment threshold?/1
  zero/1 -> Reached recruitment threshold?/3

== system FinalSim/Tricep Model/Tricep Group/Recruitment/Type F Motor Unit 3 ==
  Activation : Inport
  Reached recruitment threshold? : Switch  Threshold=0.8
  determine frequency : Fcn  Expr=((2-0.5)/(1-(0.8)))*(u(1)-(0.8))+0.5
  zero : Constant  Value=0
  Frequency (f0.5) : Outport
  wires:
  Activation/1 -> Reached recruitment threshold?/2, determine frequency/1
  Reached recruitment threshold?/1 -> Frequency (f0.5)/1
  determine frequency/1 -> Reached recruitment threshold?/1
  zero/1 -> Reached recruitment threshold?/3

== system FinalSim/Tricep Model/Tricep Group/Recruitment/Type S Motor Unit 1 ==
  Activation : Inport
  Reached recruitment threshold? : Switch  Threshold=0.17143
  determine frequency : Fcn  Expr=((2-0.5)/(1-(0.17143)))*(u(1)-(0.17143))+0.5
  zero : Constant  Value=0
  Frequency (f0.5) : Outport
  wires:
  Activation/1 -> Reached recruitment threshold?/2, determine frequency/1
  Reached recruitment threshold?/1 -> Frequency (f0.5)/1
  determine frequency/1 -> Reached recruitment threshold?/1
  zero/1 -> Reached recruitment threshold?/3

== system FinalSim/Tricep Model/Tricep Group/Recruitment/Type S Motor Unit 2 ==
  Activation : Inport
  Reached recruitment threshold? : Switch  Threshold=0.4
  determine frequency : Fcn  Expr=((2-0.5)/(1-(0.4)))*(u(1)-(0.4))+0.5
  zero : Constant  Value=0
  Frequency (f0.5) : Outport
  wires:
  Activation/1 -> Reached recruitment threshold?/2, determine frequency/1
  Reached recruitment threshold?/1 -> Frequency (f0.5)/1
  determine frequency/1 -> Reached recruitment threshold?/1
  zero/1 -> Reached recruitment threshold?/3

== system FinalSim/Tricep Model/Tricep Group/fascicles (CE & PE)/Type F Motor Units ==
  fenv : Inport
  V,L : Inport  Port=2
  Fpe2 : Inport  Port=3
  Af*(FL*FV+PE2) : Product  InputSameDT=on  RndMeth=Zero  SaturateOnIntegerOverflow=on  OutDataTypeStr=Inherit: Same as first input
  Constant : Constant
  Demux all Units : Demux  Outputs=3
      settings: DisplayOption=none
  FL : Fcn  Expr=exp(-abs((u^1.55-1)/0.74633)^2.12)
  FL*FV : Product  InputSameDT=on  RndMeth=Zero  SaturateOnIntegerOverflow=on  OutDataTypeStr=Inherit: Same as first input
  FV (lengthen) : Fcn  Expr=(0.68637-(-1.53+0*u(2)+0*u(2)^2)*u(1))/(0.68637+u(1))
  FV (shorten) : Fcn  Expr=(-9.1516-u(1))/(-9.1516+(-5.7+9.18*u(2))*u(1))
  Motor Unit 1 : Subsystem
  Motor Unit 2 : Subsystem
  Motor Unit 3 : Subsystem
  PCSA 1 : Gain  Gain=0.13333  SaturateOnIntegerOverflow=on  OutDataTypeStr=Inherit: Same as input  ParamDataTypeStr=Inherit: Same as input
  PCSA 2 : Gain  Gain=0.16667  SaturateOnIntegerOverflow=on  OutDataTypeStr=Inherit: Same as input  ParamDataTypeStr=Inherit: Same as input
  PCSA 3 : Gain  Gain=0.2  SaturateOnIntegerOverflow=on  OutDataTypeStr=Inherit: Same as input  ParamDataTypeStr=Inherit: Same as input
  PE+FL*FV : Sum  InputSameDT=on  SaturateOnIntegerOverflow=on  OutDataTypeStr=Inherit: Same as first input
  Sum all Units : Sum  Inputs=+++  InputSameDT=on  SaturateOnIntegerOverflow=on  OutDataTypeStr=Inherit: Same as first input
  Y,L : Mux  Inputs=2
  split V,L : Demux  Outputs=2
      settings: DisplayOption=none
  v > 0? : Switch
  F (Fo) : Outport
  wires:
  Constant/1 -> Y,L/1
  Y,L/1 -> Motor Unit 1/2(Y,L), Motor Unit 2/2(Y,L), Motor Unit 3/2(Y,L)
  Demux all Units/1 -> Motor Unit 1/1(fenv)
  Motor Unit 1/1(A) -> PCSA 1/1
  PCSA 1/1 -> Sum all Units/1
  Demux all Units/2 -> Motor Unit 2/1(fenv)
  Motor Unit 2/1(A) -> PCSA 2/1
  PCSA 2/1 -> Sum all Units/2
  Demux all Units/3 -> Motor Unit 3/1(fenv)
  Motor Unit 3/1(A) -> PCSA 3/1
  PCSA 3/1 -> Sum all Units/3
  Fpe2/1 -> PE+FL*FV/1
  V,L/1 -> FV (lengthen)/1, FV (shorten)/1, split V,L/1
  FV (lengthen)/1 -> v > 0?/1
  FV (shorten)/1 -> v > 0?/3
  split V,L/2 -> FL/1, Y,L/2
  FL/1 -> FL*FV/2
  split V,L/1 -> v > 0?/2
  v > 0?/1 -> FL*FV/1
  FL*FV/1 -> PE+FL*FV/2
  PE+FL*FV/1 -> Af*(FL*FV+PE2)/1
  fenv/1 -> Demux all Units/1
  Sum all Units/1 -> Af*(FL*FV+PE2)/2
  Af*(FL*FV+PE2)/1 -> F (Fo)/1

== system FinalSim/Tricep Model/Tricep Group/fascicles (CE & PE)/Type S Motor Units ==
  fenv : Inport
  V,L : Inport  Port=2
  Fpe2 : Inport  Port=3
  1/Ty : Gain  Gain=5  SaturateOnIntegerOverflow=on  OutDataTypeStr=Inherit: Same as input  ParamDataTypeStr=Inherit: Same as input
  Af*(FL*FV+PE2) : Product  InputSameDT=on  RndMeth=Zero  SaturateOnIntegerOverflow=on  OutDataTypeStr=Inherit: Same as first input
  Demux all Units : Demux  Outputs=2
      settings: DisplayOption=none
  FL : Fcn  Expr=exp(-abs((u^2.3-1)/1.1244)^1.62)
  FL*FV : Product  InputSameDT=on  RndMeth=Zero  SaturateOnIntegerOverflow=on  OutDataTypeStr=Inherit: Same as first input
  FV (lengthen) : Fcn  Expr=(0.34936-(-4.7+8.41*u(2)+-5.31*u(2)^2)*u(1))/(0.34936+u(1))
  FV (shorten) : Fcn  Expr=(-7.88-u(1))/(-7.88+(5.88+0*u(2))*u(1))
  Motor Unit 1 : Subsystem
  Motor Unit 2 : Subsystem
  PCSA 1 : Gain  Gain=0.21429  SaturateOnIntegerOverflow=on  OutDataTypeStr=Inherit: Same as input  ParamDataTypeStr=Inherit: Same as input
  PCSA 2 : Gain  Gain=0.28571  SaturateOnIntegerOverflow=on  OutDataTypeStr=Inherit: Same as input  ParamDataTypeStr=Inherit: Same as input
  PE+FL*FV : Sum  InputSameDT=on  SaturateOnIntegerOverflow=on  OutDataTypeStr=Inherit: Same as first input
  Sum all Units : Sum  InputSameDT=on  SaturateOnIntegerOverflow=on  OutDataTypeStr=Inherit: Same as first input
  Y,L : Mux  Inputs=2
  newY-oldY : Sum  Inputs=+-  InputSameDT=on  SaturateOnIntegerOverflow=on  OutDataTypeStr=Inherit: Same as first input
  split V,L : Demux  Outputs=2
      settings: DisplayOption=none
  v > 0? : Switch
  y'->y : Integrator  InitialCondition=1
  yield : Fcn  Expr=1-0.35*(1-exp(-abs(u)/0.1))
  F (Fo) : Outport
  wires:
  split V,L/1 -> yield/1, v > 0?/2
  yield/1 -> newY-oldY/1
  newY-oldY/1 -> 1/Ty/1
  1/Ty/1 -> y'->y/1
  y'->y/1 -> newY-oldY/2, Y,L/1
  Y,L/1 -> Motor Unit 1/2(Y,L), Motor Unit 2/2(Y,L)
  Demux all Units/1 -> Motor Unit 1/1(fenv)
  Motor Unit 1/1(A) -> PCSA 1/1
  PCSA 1/1 -> Sum all Units/1
  Demux all Units/2 -> Motor Unit 2/1(fenv)
  Motor Unit 2/1(A) -> PCSA 2/1
  PCSA 2/1 -> Sum all Units/2
  Fpe2/1 -> PE+FL*FV/1
  V,L/1 -> FV (lengthen)/1, FV (shorten)/1, split V,L/1
  FV (lengthen)/1 -> v > 0?/1
  FV (shorten)/1 -> v > 0?/3
  split V,L/2 -> FL/1, Y,L/2
  FL/1 -> FL*FV/2
  v > 0?/1 -> FL*FV/1
  FL*FV/1 -> PE+FL*FV/2
  PE+FL*FV/1 -> Af*(FL*FV+PE2)/1
  fenv/1 -> Demux all Units/1
  Sum all Units/1 -> Af*(FL*FV+PE2)/2
  Af*(FL*FV+PE2)/1 -> F (Fo)/1
